simulink model "red_caotica_simulink"  (R2026a)
settings: Solver=VariableStepAuto
values from neighbouring files (symbols this model uses):
  X0 = zeros(N*n,1)    [main_red_caotica.m]    (also in parametros_red.m)
settings Model: Creator=Josue Santana Robled  LastModifiedBy=Josue Santana Robled

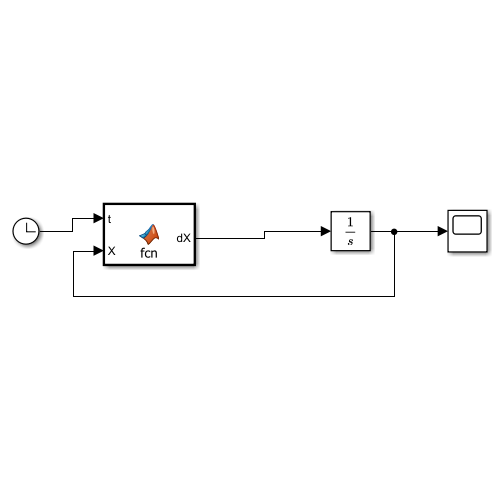
[thumbnail: Simulink's stored preview of the top-level diagram]
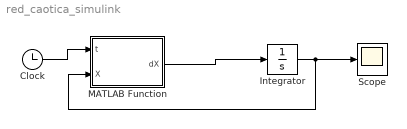
== system red_caotica_simulink ==
  Clock : Clock
  Integrator : Integrator  InitialCondition=X0
  MATLAB Function : MATLAB Function  TreatAsAtomicUnit=on
  Scope : Scope
  wires:
  Clock/1 -> MATLAB Function/1(t)
  MATLAB Function/1(dX) -> Integrator/1
  Integrator/1 -> MATLAB Function/2(X), Scope/1

== matlab function red_caotica_simulink/MATLAB Function ==
  data: t input; dX output; X input
function dX = fcn(t, X)
%#codegen

% Variables del workspace de MATLAB
N = evalin('base','N');
n = evalin('base','n');
c = evalin('base','c');
A = evalin('base','A');
W0 = evalin('base','W0');
Gamma = evalin('base','Gamma');
nodeTypes = evalin('base','nodeTypes');
nonlinear_coupling = evalin('base','nonlinear_coupling');
time_varying_weights = evalin('base','time_varying_weights');

dX = zeros(N*n,1);

% Pesos variables
if time_varying_weights
    alpha = 0.3;
    omega = 1.0;
    W = W0 .* (1 + alpha*sin(omega*t));
else
    W = W0;
end

W = (W + W')/2;
W = W .* A;

for i = 1:N
    idx_i = (i-1)*n + (1:n);
    xi = X(idx_i);

    % Dinamica interna
    if nodeTypes(i) == 1
        % Lorenz
        sigma = 10;
        rho = 28;
        beta = 8/3;
        fi = [ sigma*(xi(2)-xi(1));
               xi(1)*(rho-xi(3)) - xi(2);
               xi(1)*xi(2) - beta*xi(3) ];
    elseif nodeTypes(i) == 2
        % Rossler
        a = 0.2;
        b = 0.2;
        cc = 5.7;
        fi = [ -xi(2)-xi(3);
                xi(1)+a*xi(2);
                b + xi(3)*(xi(1)-cc) ];
    else
        fi = zeros(3,1);
    end

    % H(x_i)
    if nonlinear_coupling
        Hi = [tanh(xi(1));
              xi(2);
              0.5*sin(xi(3))];
    else
        Hi = xi;
    end

    coupling_sum = zeros(n,1);

    for j = 1:N
        if A(i,j) ~= 0
            idx_j = (j-1)*n + (1:n);
            xj = X(idx_j);

            if nonlinear_coupling
                Hj = [tanh(xj(1));
                      xj(2);
                      0.5*sin(xj(3))];
            else
                Hj = xj;
            end

            coupling_sum = coupling_sum + W(i,j) * Gamma * (Hj - Hi);
        end
    end

    dX(idx_i) = fi + c*coupling_sum;
end
